simulink model "TrainingTracerVer1"  (R2024a)
settings: Solver=FixedStepAuto  StartTime=0.0  StopTime=inf  RelTol=1e-3  EnableMultiTasking=on
undefined symbols (not defined in the file): bits
libraries: stm32blockslib x30, stm32f4xxblockslib x10, svdutilitieslib x10, simulink x5
settings Model: Creator=niijima  LastModifiedBy=niijima
settings OptimizationCC: EnhancedBackFolding=on  PassReuseOutputArgsAs=Individual arguments  ZeroExternalMemoryAtStartup=off  ZeroInternalMemoryAtStartup=off  MaxStackSize=64  OptimizeBlockOrder=speed  DifferentSizesBufferReuse=on  OptimizationCustomize=off  EfficientTunableParamExpr=on
settings DebuggingCC: ParameterTunabilityLossMsg=error
settings HardwareCC: ProdBitPerPointer=32  ProdBitPerSizeT=32  ProdBitPerPtrDiffT=32  ProdLargestAtomicInteger=Long  ProdLargestAtomicFloat=Double  ProdWordSize=32  ProdLongLongMode=on  ProdHWDeviceType=ARM Compatible->ARM Cortex-M
settings SFSimCC: MATLABDynamicMemAlloc=off
settings RTWCC: Description=Embedded Coder  SystemTargetFile=ert.tlc  HardwareBoard=STM32F3xx Based  TemplateMakefile=ert_default_tmf  Toolchain=GNU Tools for ARM Embedded Processors  BuildConfiguration=Faster Runs
settings CodeAppCC: ForceParamTrailComments=on  IgnoreCustomStorageClasses=off  OperatorAnnotations=on  SimulinkDataObjDesc=on  SFDataObjDesc=on  InsertBlockDesc=on
settings ERTTargetCC: TargetLangStandard=C99 (ISO)  CodeReplacementLibrary=ARM Cortex-M  SupportContinuousTime=on  ExtModeTransport=3  ExtModeStaticAlloc=on  ExtModeStaticAllocSize=2048  ExtModeMexFile=ext_xcp  ExtModeIntrfLevel=Level2 - Open

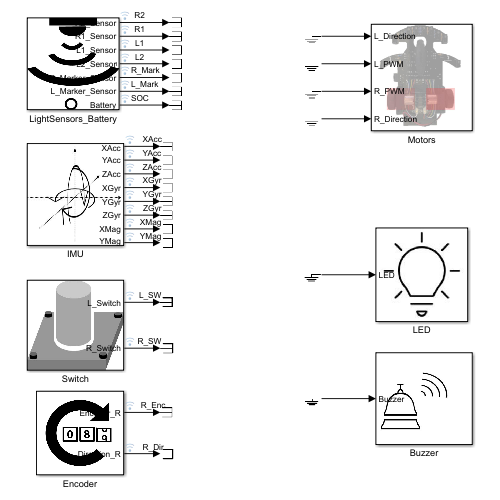
[thumbnail: Simulink's stored preview of the top-level diagram]
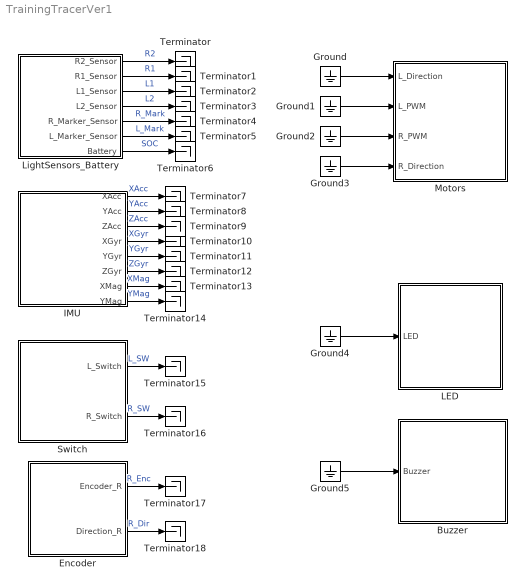
== system TrainingTracerVer1 ==
  Buzzer : Subsystem
      mask Display: image('Buzzer.jpg');
  Encoder : Subsystem
      mask Display: image('Encoder.jpg');
  Ground{,1..5} (6 alike) : Ground
  IMU : Subsystem
      mask Display: image('gyro.jpg');
  LED : Subsystem
      mask Display: image('LED.jpg');
  LightSensors_Battery : Subsystem
      mask Display: image('Sensor.jpg');
  Motors : Subsystem
      mask Display: image('Motor.jpg');
  Switch : Subsystem
      mask Display: image('Switch.jpg');
  Terminator{,1..18} (19 alike) : Terminator
  wires:
  Encoder/2(Direction_R) -> Terminator18/1  "R_Dir"
  Encoder/1(Encoder_R) -> Terminator17/1  "R_Enc"
  IMU/8(YMag) -> Terminator14/1  "YMag"
  IMU/7(XMag) -> Terminator13/1  "XMag"
  IMU/6(ZGyr) -> Terminator12/1  "ZGyr"
  IMU/5(YGyr) -> Terminator11/1  "YGyr"
  IMU/4(XGyr) -> Terminator10/1  "XGyr"
  IMU/3(ZAcc) -> Terminator9/1  "ZAcc"
  IMU/2(YAcc) -> Terminator8/1  "YAcc"
  IMU/1(XAcc) -> Terminator7/1  "XAcc"
  LightSensors_Battery/7(Battery) -> Terminator6/1  "SOC"
  LightSensors_Battery/6(L_Marker_Sensor) -> Terminator5/1  "L_Mark"
  LightSensors_Battery/5(R_Marker_Sensor) -> Terminator4/1  "R_Mark"
  LightSensors_Battery/4(L2_Sensor) -> Terminator3/1  "L2"
  LightSensors_Battery/3(L1_Sensor) -> Terminator2/1  "L1"
  LightSensors_Battery/2(R1_Sensor) -> Terminator1/1  "R1"
  LightSensors_Battery/1(R2_Sensor) -> Terminator/1  "R2"
  Ground3/1 -> Motors/4(R_Direction)
  Ground1/1 -> Motors/2(L_PWM)
  Ground5/1 -> Buzzer/1(Buzzer)
  Ground4/1 -> LED/1(LED)
  Ground2/1 -> Motors/3(R_PWM)
  Ground/1 -> Motors/1(L_Direction)
  Switch/1(L_Switch) -> Terminator15/1  "L_SW"
  Switch/2(R_Switch) -> Terminator16/1  "R_SW"

== system TrainingTracerVer1/Buzzer ==
  Buzzer : Inport
  Buzzer_ : stm32f4xxblockslib/Digital Port Write  PortName=GPIOA  PinNumber=[12]  ReadOperation=off  IOAsArray=on  EnableSimPort=off
      settings: LibrarySourceBlock=stm32f3xxblockslib/Digital Port Write
  wires:
  Buzzer/1 -> Buzzer_/1

== system TrainingTracerVer1/Encoder ==
  Encoder_Left : stm32blockslib/Encoder  Commented=on  TimerModule=TIM20  EnableResetInput=off  OutputDirection=on  SampleTime=-1
      settings: LibrarySourceBlock=stm32f3xxblockslib/Encoder
  Encoder_Right : stm32blockslib/Encoder  TimerModule=TIM2  EnableResetInput=off  OutputDirection=on  SampleTime=-1
      settings: LibrarySourceBlock=stm32f3xxblockslib/Encoder
  Terminator : Terminator
  Terminator1 : Terminator
  Encoder_R : Outport
  Direction_R : Outport  Port=2
  wires:
  Encoder_Right/2 -> Direction_R/1  "Direction_R"
  Encoder_Right/1 -> Encoder_R/1  "Encoder_R"
  Encoder_Left/1 -> Terminator/1  "Encoder_L"
  Encoder_Left/2 -> Terminator1/1  "Direction_L"

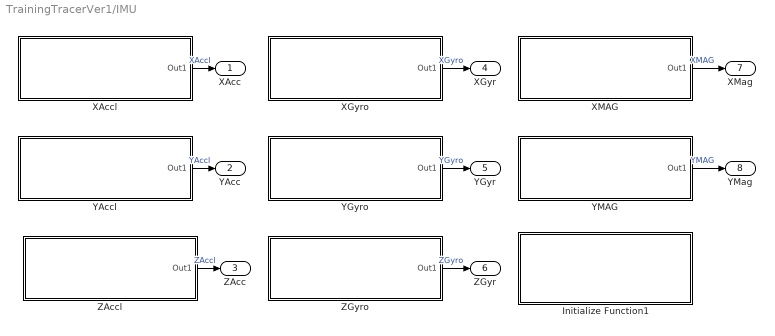
== system TrainingTracerVer1/IMU ==
  Initialize Function1 : Subsystem  TreatAsAtomicUnit=on
  XAccl : Subsystem
  XGyro : Subsystem
  XMAG : Subsystem
  YAccl : Subsystem
  YGyro : Subsystem
  YMAG : Subsystem
  ZAccl : Subsystem
  ZGyro : Subsystem
  XAcc : Outport
  YAcc : Outport  Port=2
  ZAcc : Outport  Port=3
  XGyr : Outport  Port=4
  YGyr : Outport  Port=5
  ZGyr : Outport  Port=6
  XMag : Outport  Port=7
  YMag : Outport  Port=8
  wires:
  XMAG/1(Out1) -> XMag/1  "XMAG"
  YGyro/1(Out1) -> YGyr/1  "YGyro"
  YMAG/1(Out1) -> YMag/1  "YMAG"
  ZGyro/1(Out1) -> ZGyr/1  "ZGyro"
  ZAccl/1(Out1) -> ZAcc/1  "ZAccl"
  XGyro/1(Out1) -> XGyr/1  "XGyro"
  YAccl/1(Out1) -> YAcc/1  "YAccl"
  XAccl/1(Out1) -> XAcc/1  "XAccl"

== system TrainingTracerVer1/LED ==
  LED : Inport
  LED_ : stm32f4xxblockslib/Digital Port Write  PortName=GPIOB  PinNumber=[3]  ReadOperation=off  IOAsArray=on  EnableSimPort=off
      settings: LibrarySourceBlock=stm32f3xxblockslib/Digital Port Write
  wires:
  LED/1 -> LED_/1

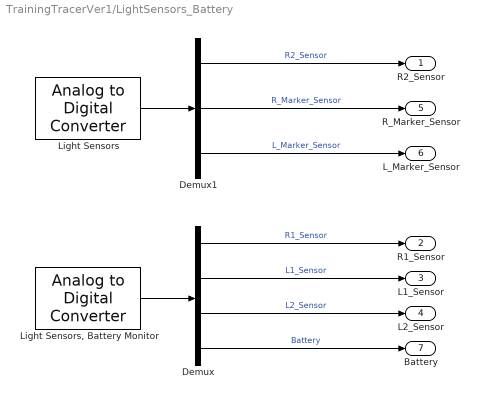
== system TrainingTracerVer1/LightSensors_Battery ==
  Demux : Demux
  Demux1 : Demux  Outputs=3
  Light Sensors : stm32f4xxblockslib/Analog to Digital Converter  ADCModule=ADC1  ConversionGroup=Regular  TriggerMode=Trigger and read  NumberOfConversions=3  EnableBufferConv=off  BufferLength=1  OutputStatus=off  SampleTime=-1  EnableSimPort=off
      settings: LibrarySourceBlock=stm32f3xxblockslib/Analog to Digital Converter
  "Light Sensors, Battery Monitor" : stm32f4xxblockslib/Analog to Digital Converter  ADCModule=ADC2  ConversionGroup=Regular  TriggerMode=Trigger and read  NumberOfConversions=4  EnableBufferConv=off  BufferLength=1  OutputStatus=off  SampleTime=-1  EnableSimPort=off
      settings: LibrarySourceBlock=stm32f3xxblockslib/Analog to Digital Converter
  R2_Sensor : Outport
  R1_Sensor : Outport  Port=2
  L1_Sensor : Outport  Port=3
  L2_Sensor : Outport  Port=4
  R_Marker_Sensor : Outport  Port=5
  L_Marker_Sensor : Outport  Port=6
  Battery : Outport  Port=7
  wires:
  Demux/2 -> L1_Sensor/1  "L1_Sensor"
  "Light Sensors, Battery Monitor"/1 -> Demux/1
  Demux1/1 -> R2_Sensor/1  "R2_Sensor"
  Light Sensors/1 -> Demux1/1
  Demux/3 -> L2_Sensor/1  "L2_Sensor"
  Demux1/3 -> L_Marker_Sensor/1  "L_Marker_Sensor"
  Demux1/2 -> R_Marker_Sensor/1  "R_Marker_Sensor"
  Demux/4 -> Battery/1  "Battery"
  Demux/1 -> R1_Sensor/1  "R1_Sensor"

== system TrainingTracerVer1/Motors ==
  L_Direction : Inport
  L_PWM : Inport  Port=2
  R_PWM : Inport  Port=3
  R_Direction : Inport  Port=4
  Left_Direction : stm32f4xxblockslib/Digital Port Write  PortName=GPIOA  PinNumber=[10]  ReadOperation=off  IOAsArray=on  EnableSimPort=off
      settings: LibrarySourceBlock=stm32f3xxblockslib/Digital Port Write
  Left_PWM : stm32f4xxblockslib/PWM Output  TimerModule=TIM1  DutycycleUnits=Percentage  EnableChannel1=off  EnableChannel2=off  EnableChannel3=off  EnableChannel4=on  EnableCounterInput=off  EnableMainOutputInput=off  EnableFrequencyInput=off  SetRCAfterCE=off  OutputDirection=off  OutputMainOutputEnableStatus=off  SampleTime=0.1  EnableSimPort=off  EnableUpdateEvent=off  EnableCaptureCompare1Event=off  EnableCaptureCompare2Event=off  EnableCaptureCompare3Event=off  EnableCaptureCompare4Event=off  EnableTriggerEvent=off  EnableBreakEvent=off  ProcessorFamily=STM32F3  hoistedMaskSrc=ECSoC/ECSimCodegen/PWM Output
      settings: LibrarySourceBlock=stm32f3xxblockslib/PWM Output
  Right_Direction : stm32f4xxblockslib/Digital Port Write  PortName=GPIOB  PinNumber=[4]  ReadOperation=off  IOAsArray=on  EnableSimPort=off
      settings: LibrarySourceBlock=stm32f3xxblockslib/Digital Port Write
  Right_PWM : stm32f4xxblockslib/PWM Output  TimerModule=TIM17  DutycycleUnits=Percentage  EnableChannel1=on  EnableChannel2=off  EnableChannel3=off  EnableChannel4=off  EnableCounterInput=off  EnableMainOutputInput=off  EnableFrequencyInput=off  SetRCAfterCE=off  OutputDirection=off  OutputMainOutputEnableStatus=off  SampleTime=0.1  EnableSimPort=off  EnableUpdateEvent=off  EnableCaptureCompare1Event=off  EnableCaptureCompare2Event=off  EnableCaptureCompare3Event=off  EnableCaptureCompare4Event=off  EnableTriggerEvent=off  EnableBreakEvent=off  ProcessorFamily=STM32F3  hoistedMaskSrc=ECSoC/ECSimCodegen/PWM Output
      settings: LibrarySourceBlock=stm32f3xxblockslib/PWM Output
  wires:
  R_Direction/1 -> Right_Direction/1
  R_PWM/1 -> Right_PWM/1
  L_Direction/1 -> Left_Direction/1
  L_PWM/1 -> Left_PWM/1

== system TrainingTracerVer1/Switch ==
  L_Switch_ : stm32f4xxblockslib/Digital Port Read  PortName=GPIOF  PinNumber=[0]  ReadOperation=on  IOAsArray=off  SampleTime=-1  EnableSimPort=off
      settings: LibrarySourceBlock=stm32f3xxblockslib/Digital Port Read
  R_Switch_ : stm32f4xxblockslib/Digital Port Read  PortName=GPIOF  PinNumber=[1]  ReadOperation=on  IOAsArray=off  SampleTime=-1  EnableSimPort=off
      settings: LibrarySourceBlock=stm32f3xxblockslib/Digital Port Read
  L_Switch : Outport
  R_Switch : Outport  Port=2
  wires:
  R_Switch_/1 -> R_Switch/1  "R_Switch"
  L_Switch_/1 -> L_Switch/1  "L_Switch"

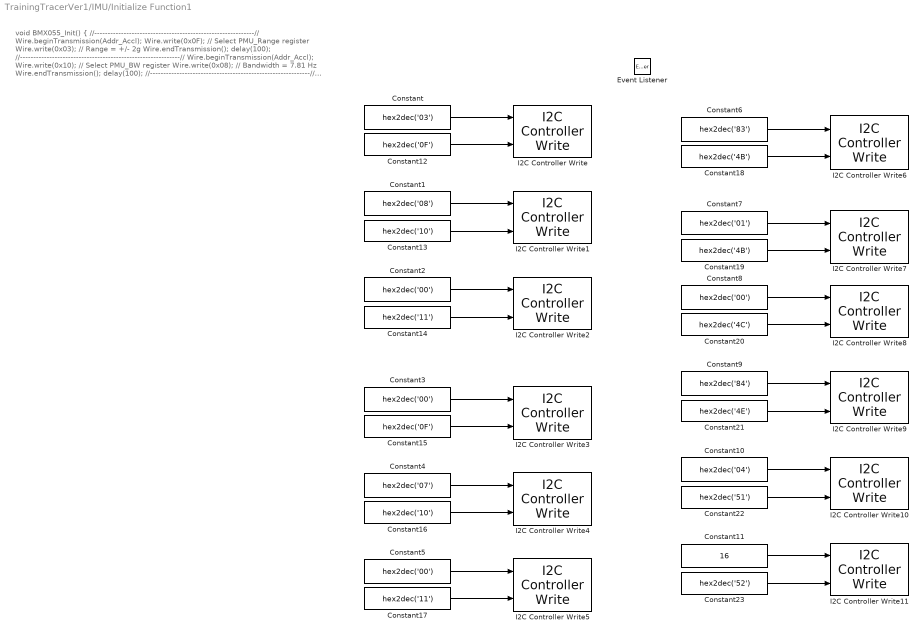
== system TrainingTracerVer1/IMU/Initialize Function1 ==
  note: void BMX055_Init()
      | { //------------------------------------------------------------//
      | Wire.beginTransmission(Addr_Accl);
      | Wire.write(0x0F); // Select PMU_Range register
      | Wire.write(0x03); // Range = +/- 2g
      | Wire.endTransmission();
      | delay(100);
      | //------------------------------------------------------------//
      | Wire.beginTransmission(Addr_Accl);
      | Wire.write(0x10); // Select PMU_BW register
      | Wire.write(0x08); // Bandwidth = 7.81 Hz
      | Wire.endTransmission();
      | delay(100);
      | //------------------------------------------------------------//
      | Wire.beginTransmission(Addr_Accl);
      | Wire.write(0x11); // Select PMU_LPW register
      | Wire.write(0x00); // Normal mode, Sleep duration = 0.5ms
      | Wire.endTransmission();
      | delay(100);
      | //------------------------------------------------------------//
      | Wire.beginTransmission(Addr_Gyro);
      | Wire.write(0x0F); // Select Range register
      | Wire.write(0x00); // Full scale = +/- 2000 degree/s
      | Wire.endTransmission();
      | delay(100);
      | //------------------------------------------------------------//
      | Wire.beginTransmission(Addr_Gyro);
      | Wire.write(0x10); // Select Bandwidth register
      | Wire.write(0x07); // ODR = 100 Hz
      | Wire.endTransmission();
      | delay(100);
      | //------------------------------------------------------------//
      | Wire.beginTransmission(Addr_Gyro);
      | Wire.write(0x11); // Select LPM1 register
      | Wire.write(0x00); // Normal mode, Sleep duration = 2ms
      | Wire.endTransmission();
      | delay(100);
      | //------------------------------------------------------------//
      | Wire.beginTransmission(Addr_Mag);
      | Wire.write(0x4B); // Select Mag register
      | Wire.write(0x83); // Soft reset
      | Wire.endTransmission();
      | delay(100);
      | //------------------------------------------------------------//
      | Wire.beginTransmission(Addr_Mag);
      | Wire.write(0x4B); // Select Mag register
      | Wire.write(0x01); // Soft reset
      | Wire.endTransmission();
      | delay(100);
      | //------------------------------------------------------------//
      | Wire.beginTransmission(Addr_Mag);
      | Wire.write(0x4C); // Select Mag register
      | Wire.write(0x00); // Normal Mode, ODR = 10 Hz
      | Wire.endTransmission();
      | //------------------------------------------------------------//
      | Wire.beginTransmission(Addr_Mag);
      | Wire.write(0x4E); // Select Mag register
      | Wire.write(0x84); // X, Y, Z-Axis enabled
      | Wire.endTransmission();
      | //------------------------------------------------------------//
      | Wire.beginTransmission(Addr_Mag);
      | Wire.write(0x51); // Select Mag register
      | Wire.write(0x04); // No. of Repetitions for X-Y Axis = 9
      | Wire.endTransmission();
      | //------------------------------------------------------------//
      | Wire.beginTransmission(Addr_Mag);
      | Wire.write(0x52); // Select Mag register
      | Wire.write(16); // No. of Repetitions for Z-Axis = 15
      | Wire.endTransmission();}
  Constant : Constant  Value=hex2dec('03')  VectorParams1D=off  OutDataTypeStr=uint8
  Constant1 : Constant  Value=hex2dec('08')  VectorParams1D=off  OutDataTypeStr=uint8
  Constant10 : Constant  Value=hex2dec('04')  VectorParams1D=off  OutDataTypeStr=uint8
  Constant11 : Constant  Value=16  VectorParams1D=off  OutDataTypeStr=uint8
  Constant12 : Constant  Value=hex2dec('0F')  OutDataTypeStr=uint8
  Constant13 : Constant  Value=hex2dec('10')  OutDataTypeStr=uint8
  Constant14 : Constant  Value=hex2dec('11')  OutDataTypeStr=uint8
  Constant15 : Constant  Value=hex2dec('0F')  OutDataTypeStr=uint8
  Constant16 : Constant  Value=hex2dec('10')  OutDataTypeStr=uint8
  Constant17 : Constant  Value=hex2dec('11')  OutDataTypeStr=uint8
  Constant18 : Constant  Value=hex2dec('4B')  OutDataTypeStr=uint8
  Constant19 : Constant  Value=hex2dec('4B')  OutDataTypeStr=uint8
  Constant{2..3,5,8} (4 alike) : Constant  Value=hex2dec('00')  VectorParams1D=off  OutDataTypeStr=uint8
  Constant20 : Constant  Value=hex2dec('4C')  OutDataTypeStr=uint8
  Constant21 : Constant  Value=hex2dec('4E')  OutDataTypeStr=uint8
  Constant22 : Constant  Value=hex2dec('51')  OutDataTypeStr=uint8
  Constant23 : Constant  Value=hex2dec('52')  OutDataTypeStr=uint8
  Constant4 : Constant  Value=hex2dec('07')  VectorParams1D=off  OutDataTypeStr=uint8
  Constant6 : Constant  Value=hex2dec('83')  VectorParams1D=off  OutDataTypeStr=uint8
  Constant7 : Constant  Value=hex2dec('01')  VectorParams1D=off  OutDataTypeStr=uint8
  Constant9 : Constant  Value=hex2dec('84')  VectorParams1D=off  OutDataTypeStr=uint8
  Event Listener : EventListener  DisableCoverage=on  EventName=reset
  I2C Controller Write : stm32blockslib/I2C Controller Write  I2CModule=I2C1  Mode=Controller  AddressingMode=7-bits  PeripheralByteOrder=LittleEndian  OwnPeripheralAddress=uint8(170)  PeripheralAddressVia=Dialog  PeripheralAddress=hex2dec('19')  RegisterAddressMode=on  RegisterAddressVia=Inport  RegisterAddress=hex2dec('0F')  RepeatedStart=off  NoAck=off  OutputStatus=off  BlockMode=Transmit  DataType=uint8  DataLength=1  Timeout=0.1  SampleTime=-1
      settings: LibrarySourceBlock=stm32f4xxblockslib/I2C Controller Write
  I2C Controller Write1 : stm32blockslib/I2C Controller Write  I2CModule=I2C1  Mode=Controller  AddressingMode=7-bits  PeripheralByteOrder=LittleEndian  OwnPeripheralAddress=uint8(170)  PeripheralAddressVia=Dialog  PeripheralAddress=hex2dec('19')  RegisterAddressMode=on  RegisterAddressVia=Inport  RegisterAddress=hex2dec('10')  RepeatedStart=off  NoAck=off  OutputStatus=off  BlockMode=Transmit  DataType=uint8  DataLength=1  Timeout=0.1  SampleTime=-1
      settings: LibrarySourceBlock=stm32f4xxblockslib/I2C Controller Write
  I2C Controller Write10 : stm32blockslib/I2C Controller Write  I2CModule=I2C1  Mode=Controller  AddressingMode=7-bits  PeripheralByteOrder=LittleEndian  OwnPeripheralAddress=uint8(170)  PeripheralAddressVia=Dialog  PeripheralAddress=hex2dec('13')  RegisterAddressMode=on  RegisterAddressVia=Inport  RegisterAddress=hex2dec('51')  RepeatedStart=off  NoAck=off  OutputStatus=off  BlockMode=Transmit  DataType=uint8  DataLength=1  Timeout=0.01  SampleTime=-1
      settings: LibrarySourceBlock=stm32f4xxblockslib/I2C Controller Write
  I2C Controller Write11 : stm32blockslib/I2C Controller Write  I2CModule=I2C1  Mode=Controller  AddressingMode=7-bits  PeripheralByteOrder=LittleEndian  OwnPeripheralAddress=uint8(170)  PeripheralAddressVia=Dialog  PeripheralAddress=hex2dec('13')  RegisterAddressMode=on  RegisterAddressVia=Inport  RegisterAddress=hex2dec('52')  RepeatedStart=off  NoAck=off  OutputStatus=off  BlockMode=Transmit  DataType=uint8  DataLength=1  Timeout=0.01  SampleTime=-1
      settings: LibrarySourceBlock=stm32f4xxblockslib/I2C Controller Write
  I2C Controller Write2 : stm32blockslib/I2C Controller Write  I2CModule=I2C1  Mode=Controller  AddressingMode=7-bits  PeripheralByteOrder=LittleEndian  OwnPeripheralAddress=uint8(170)  PeripheralAddressVia=Dialog  PeripheralAddress=hex2dec('19')  RegisterAddressMode=on  RegisterAddressVia=Inport  RegisterAddress=hex2dec('11')  RepeatedStart=off  NoAck=off  OutputStatus=off  BlockMode=Transmit  DataType=uint8  DataLength=1  Timeout=0.1  SampleTime=-1
      settings: LibrarySourceBlock=stm32f4xxblockslib/I2C Controller Write
  I2C Controller Write3 : stm32blockslib/I2C Controller Write  I2CModule=I2C1  Mode=Controller  AddressingMode=7-bits  PeripheralByteOrder=LittleEndian  OwnPeripheralAddress=uint8(170)  PeripheralAddressVia=Dialog  PeripheralAddress=hex2dec('69')  RegisterAddressMode=on  RegisterAddressVia=Inport  RegisterAddress=hex2dec('0F')  RepeatedStart=off  NoAck=off  OutputStatus=off  BlockMode=Transmit  DataType=uint8  DataLength=1  Timeout=0.1  SampleTime=-1
      settings: LibrarySourceBlock=stm32f4xxblockslib/I2C Controller Write
  I2C Controller Write4 : stm32blockslib/I2C Controller Write  I2CModule=I2C1  Mode=Controller  AddressingMode=7-bits  PeripheralByteOrder=LittleEndian  OwnPeripheralAddress=uint8(170)  PeripheralAddressVia=Dialog  PeripheralAddress=hex2dec('69')  RegisterAddressMode=on  RegisterAddressVia=Inport  RegisterAddress=hex2dec('10')  RepeatedStart=off  NoAck=off  OutputStatus=off  BlockMode=Transmit  DataType=uint8  DataLength=1  Timeout=0.1  SampleTime=-1
      settings: LibrarySourceBlock=stm32f4xxblockslib/I2C Controller Write
  I2C Controller Write5 : stm32blockslib/I2C Controller Write  I2CModule=I2C1  Mode=Controller  AddressingMode=7-bits  PeripheralByteOrder=LittleEndian  OwnPeripheralAddress=uint8(170)  PeripheralAddressVia=Dialog  PeripheralAddress=hex2dec('69')  RegisterAddressMode=on  RegisterAddressVia=Inport  RegisterAddress=hex2dec('11')  RepeatedStart=off  NoAck=off  OutputStatus=off  BlockMode=Transmit  DataType=uint8  DataLength=1  Timeout=0.1  SampleTime=-1
      settings: LibrarySourceBlock=stm32f4xxblockslib/I2C Controller Write
  I2C Controller Write6 : stm32blockslib/I2C Controller Write  I2CModule=I2C1  Mode=Controller  AddressingMode=7-bits  PeripheralByteOrder=LittleEndian  OwnPeripheralAddress=uint8(170)  PeripheralAddressVia=Dialog  PeripheralAddress=hex2dec('13')  RegisterAddressMode=on  RegisterAddressVia=Inport  RegisterAddress=hex2dec('4B')  RepeatedStart=off  NoAck=off  OutputStatus=off  BlockMode=Transmit  DataType=uint8  DataLength=1  Timeout=0.1  SampleTime=-1
      settings: LibrarySourceBlock=stm32f4xxblockslib/I2C Controller Write
  I2C Controller Write7 : stm32blockslib/I2C Controller Write  I2CModule=I2C1  Mode=Controller  AddressingMode=7-bits  PeripheralByteOrder=LittleEndian  OwnPeripheralAddress=uint8(170)  PeripheralAddressVia=Dialog  PeripheralAddress=hex2dec('13')  RegisterAddressMode=on  RegisterAddressVia=Inport  RegisterAddress=hex2dec('4B')  RepeatedStart=off  NoAck=off  OutputStatus=off  BlockMode=Transmit  DataType=uint8  DataLength=1  Timeout=0.1  SampleTime=-1
      settings: LibrarySourceBlock=stm32f4xxblockslib/I2C Controller Write
  I2C Controller Write8 : stm32blockslib/I2C Controller Write  I2CModule=I2C1  Mode=Controller  AddressingMode=7-bits  PeripheralByteOrder=LittleEndian  OwnPeripheralAddress=uint8(170)  PeripheralAddressVia=Dialog  PeripheralAddress=hex2dec('13')  RegisterAddressMode=on  RegisterAddressVia=Inport  RegisterAddress=hex2dec('4C')  RepeatedStart=off  NoAck=off  OutputStatus=off  BlockMode=Transmit  DataType=uint8  DataLength=1  Timeout=0.01  SampleTime=-1
      settings: LibrarySourceBlock=stm32f4xxblockslib/I2C Controller Write
  I2C Controller Write9 : stm32blockslib/I2C Controller Write  I2CModule=I2C1  Mode=Controller  AddressingMode=7-bits  PeripheralByteOrder=LittleEndian  OwnPeripheralAddress=uint8(170)  PeripheralAddressVia=Dialog  PeripheralAddress=hex2dec('13')  RegisterAddressMode=on  RegisterAddressVia=Inport  RegisterAddress=hex2dec('4E')  RepeatedStart=off  NoAck=off  OutputStatus=off  BlockMode=Transmit  DataType=uint8  DataLength=1  Timeout=0.01  SampleTime=-1
      settings: LibrarySourceBlock=stm32f4xxblockslib/I2C Controller Write
  wires:
  Constant/1 -> I2C Controller Write/1
  Constant1/1 -> I2C Controller Write1/1
  Constant2/1 -> I2C Controller Write2/1
  Constant5/1 -> I2C Controller Write5/1
  Constant4/1 -> I2C Controller Write4/1
  Constant3/1 -> I2C Controller Write3/1
  Constant6/1 -> I2C Controller Write6/1
  Constant7/1 -> I2C Controller Write7/1
  Constant8/1 -> I2C Controller Write8/1
  Constant9/1 -> I2C Controller Write9/1
  Constant10/1 -> I2C Controller Write10/1
  Constant11/1 -> I2C Controller Write11/1
  Constant12/1 -> I2C Controller Write/2
  Constant13/1 -> I2C Controller Write1/2
  Constant14/1 -> I2C Controller Write2/2
  Constant15/1 -> I2C Controller Write3/2
  Constant16/1 -> I2C Controller Write4/2
  Constant17/1 -> I2C Controller Write5/2
  Constant18/1 -> I2C Controller Write6/2
  Constant19/1 -> I2C Controller Write7/2
  Constant20/1 -> I2C Controller Write8/2
  Constant21/1 -> I2C Controller Write9/2
  Constant22/1 -> I2C Controller Write10/2
  Constant23/1 -> I2C Controller Write11/2

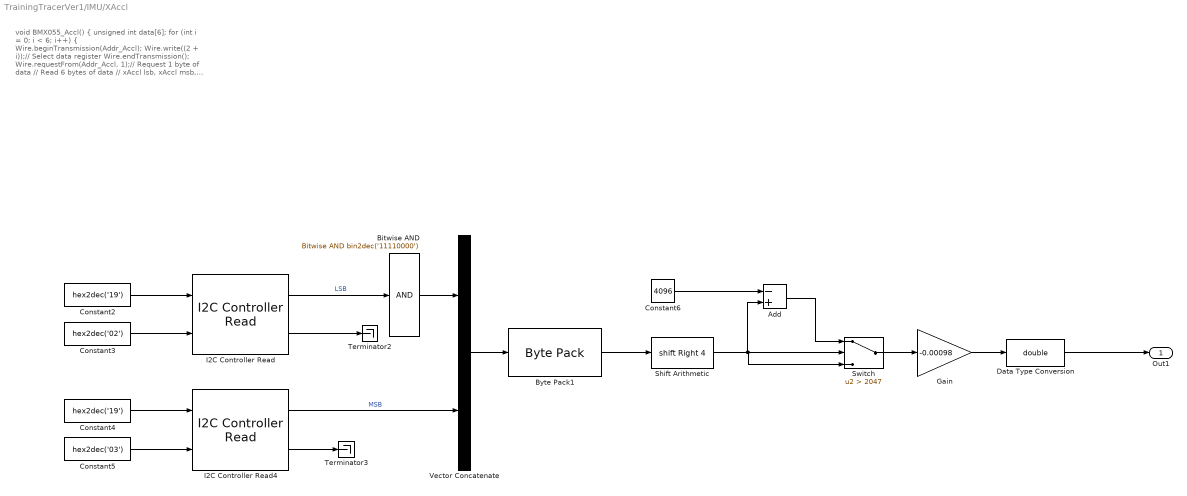
== system TrainingTracerVer1/IMU/XAccl ==
  note: void BMX055_Accl()
      | {
      | unsigned int data[6];
      | for (int i = 0; i < 6; i++)
      | {
      | Wire.beginTransmission(Addr_Accl);
      | Wire.write((2 + i));// Select data register
      | Wire.endTransmission();
      | Wire.requestFrom(Addr_Accl, 1);// Request 1 byte of data
      | // Read 6 bytes of data
      | // xAccl lsb, xAccl msb, yAccl lsb, yAccl msb, zAccl lsb, zAccl msb
      | if (Wire.available() == 1)
      | data[i] = Wire.read();
      | }
      | // Convert the data to 12-bits
      | xAccl = ((data[1] * 256) + (data[0] & 0xF0)) / 16;
      | if (xAccl > 2047) xAccl -= 4096;
      | xAccl = xAccl * 0.00098; // range = +/-2g
      | }
  Add : Sum  Inputs=-+
  Bitwise AND : simulink/Logic and Bit Operations/Bitwise Operator  logicop=AND  UseBitMask=on  BitMask=bin2dec('11110000')  BitMaskRealWorld=Stored Integer
      settings: LibrarySourceBlock=|
      | simulink/Quick Insert/Logic and Bit
      | Operations/Bitwise AND
  Byte Pack1 : svdutilitieslib/Byte Pack  maskPackedDataType=uint16  datatypes={'uint8'}  byteAlign=1  blockPlatform=arduinoert
      settings: LibrarySourceBlock=mcblib/Signal Management/Byte Pack
  Constant2 : Constant  Value=hex2dec('19')  OutDataTypeStr=uint8
  Constant3 : Constant  Value=hex2dec('02')  OutDataTypeStr=uint8
  Constant4 : Constant  Value=hex2dec('19')  OutDataTypeStr=uint8
  Constant5 : Constant  Value=hex2dec('03')  OutDataTypeStr=uint8
  Constant6 : Constant  Value=4096
  Data Type Conversion : DataTypeConversion  OutDataTypeStr=double  SaturateOnIntegerOverflow=off  RndMeth=Floor
  Gain : Gain  Gain=-0.00098
  I2C Controller Read : stm32blockslib/I2C Controller Read  I2CModule=I2C1  Mode=Controller  AddressingMode=7-bits  PeripheralByteOrder=LittleEndian  OwnPeripheralAddress=uint8(170)  PeripheralAddressVia=Inport  PeripheralAddress=0x19  RegisterAddressMode=on  RegisterAddressVia=Inport  RegisterAddress=0x02  RepeatedStart=off  NoAck=off  OutputStatus=on  BlockMode=Receive  DataType=uint8  DataLength=1  Timeout=0.1  SampleTime=-1
      settings: LibrarySourceBlock=stm32f4xxblockslib/I2C Controller Read
  I2C Controller Read4 : stm32blockslib/I2C Controller Read  I2CModule=I2C1  Mode=Controller  AddressingMode=7-bits  PeripheralByteOrder=LittleEndian  OwnPeripheralAddress=uint8(170)  PeripheralAddressVia=Inport  PeripheralAddress=0x19  RegisterAddressMode=on  RegisterAddressVia=Inport  RegisterAddress=0x02  RepeatedStart=off  NoAck=off  OutputStatus=on  BlockMode=Receive  DataType=uint8  DataLength=1  Timeout=0.1  SampleTime=-1
      settings: LibrarySourceBlock=stm32f4xxblockslib/I2C Controller Read
  Shift Arithmetic : ArithShift  BitShiftNumber=4  BitShiftDirection=Right
  Switch : Switch  Criteria=u2 > Threshold  Threshold=2047  SaturateOnIntegerOverflow=off  InputSameDT=off
  Terminator2 : Terminator
  Terminator3 : Terminator
  Vector Concatenate : Concatenate
  Out1 : Outport
  wires:
  Constant3/1 -> I2C Controller Read/2
  Add/1 -> Switch/1
  Constant4/1 -> I2C Controller Read4/1
  Byte Pack1/1 -> Shift Arithmetic/1
  Gain/1 -> Data Type Conversion/1
  I2C Controller Read/2 -> Terminator2/1
  Constant2/1 -> I2C Controller Read/1
  Shift Arithmetic/1 -> Switch/2, Switch/3, Add/2
  Bitwise AND/1 -> Vector Concatenate/1
  Constant6/1 -> Add/1
  I2C Controller Read4/2 -> Terminator3/1
  I2C Controller Read4/1 -> Vector Concatenate/2  "MSB"
  Constant5/1 -> I2C Controller Read4/2
  Switch/1 -> Gain/1
  I2C Controller Read/1 -> Bitwise AND/1  "LSB"
  Vector Concatenate/1 -> Byte Pack1/1
  Data Type Conversion/1 -> Out1/1

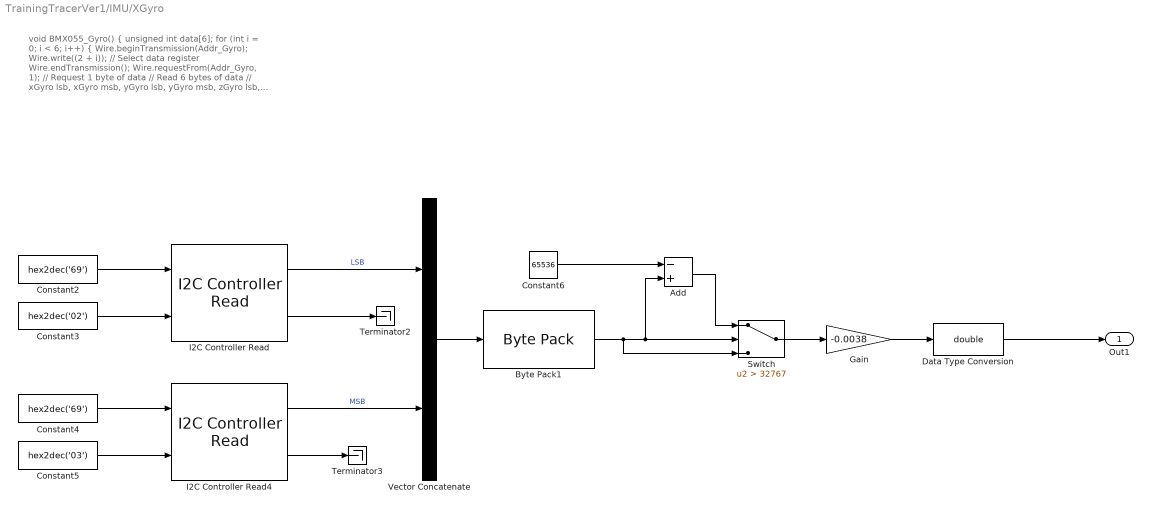
== system TrainingTracerVer1/IMU/XGyro ==
  note: void BMX055_Gyro()
      | {
      | unsigned int data[6];
      | for (int i = 0; i < 6; i++)
      | {
      | Wire.beginTransmission(Addr_Gyro);
      | Wire.write((2 + i)); // Select data register
      | Wire.endTransmission();
      | Wire.requestFrom(Addr_Gyro, 1); // Request 1 byte of data
      | // Read 6 bytes of data
      | // xGyro lsb, xGyro msb, yGyro lsb, yGyro msb, zGyro lsb, zGyro msb
      | if (Wire.available() == 1)
      | data[i] = Wire.read();
      | }
      | // Convert the data
      | xGyro = (data[1] * 256) + data[0];
      | if (xGyro > 32767) xGyro -= 65536;
      | }
  Add : Sum  Inputs=-+
  Byte Pack1 : svdutilitieslib/Byte Pack  maskPackedDataType=uint16  datatypes={'uint8'}  byteAlign=1  blockPlatform=arduinoert
      settings: LibrarySourceBlock=mcblib/Signal Management/Byte Pack
  Constant2 : Constant  Value=hex2dec('69')  OutDataTypeStr=uint8
  Constant3 : Constant  Value=hex2dec('02')  OutDataTypeStr=uint8
  Constant4 : Constant  Value=hex2dec('69')  OutDataTypeStr=uint8
  Constant5 : Constant  Value=hex2dec('03')  OutDataTypeStr=uint8
  Constant6 : Constant  Value=65536
  Data Type Conversion : DataTypeConversion  OutDataTypeStr=double  SaturateOnIntegerOverflow=off  RndMeth=Floor
  Gain : Gain  Gain=-0.0038
  I2C Controller Read : stm32blockslib/I2C Controller Read  I2CModule=I2C1  Mode=Controller  AddressingMode=7-bits  PeripheralByteOrder=LittleEndian  OwnPeripheralAddress=uint8(170)  PeripheralAddressVia=Inport  PeripheralAddress=0x19  RegisterAddressMode=on  RegisterAddressVia=Inport  RegisterAddress=0x02  RepeatedStart=off  NoAck=off  OutputStatus=on  BlockMode=Receive  DataType=uint8  DataLength=1  Timeout=0.1  SampleTime=-1
      settings: LibrarySourceBlock=stm32f4xxblockslib/I2C Controller Read
  I2C Controller Read4 : stm32blockslib/I2C Controller Read  I2CModule=I2C1  Mode=Controller  AddressingMode=7-bits  PeripheralByteOrder=LittleEndian  OwnPeripheralAddress=uint8(170)  PeripheralAddressVia=Inport  PeripheralAddress=0x19  RegisterAddressMode=on  RegisterAddressVia=Inport  RegisterAddress=0x02  RepeatedStart=off  NoAck=off  OutputStatus=on  BlockMode=Receive  DataType=uint8  DataLength=1  Timeout=0.1  SampleTime=-1
      settings: LibrarySourceBlock=stm32f4xxblockslib/I2C Controller Read
  Switch : Switch  Criteria=u2 > Threshold  Threshold=32767  SaturateOnIntegerOverflow=off  InputSameDT=off
  Terminator2 : Terminator
  Terminator3 : Terminator
  Vector Concatenate : Concatenate
  Out1 : Outport
  wires:
  Constant3/1 -> I2C Controller Read/2
  Add/1 -> Switch/1
  Constant4/1 -> I2C Controller Read4/1
  Gain/1 -> Data Type Conversion/1
  I2C Controller Read/2 -> Terminator2/1
  Constant2/1 -> I2C Controller Read/1
  Byte Pack1/1 -> Switch/2, Add/2, Switch/3
  Constant6/1 -> Add/1
  I2C Controller Read4/2 -> Terminator3/1
  I2C Controller Read4/1 -> Vector Concatenate/2  "MSB"
  Constant5/1 -> I2C Controller Read4/2
  Switch/1 -> Gain/1
  I2C Controller Read/1 -> Vector Concatenate/1  "LSB"
  Vector Concatenate/1 -> Byte Pack1/1
  Data Type Conversion/1 -> Out1/1

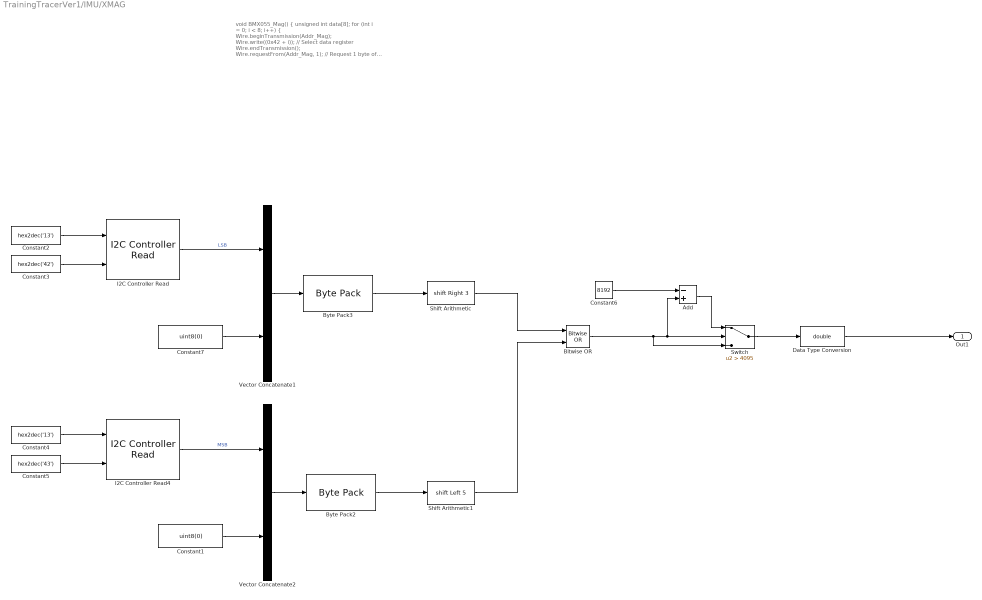
== system TrainingTracerVer1/IMU/XMAG ==
  note: void BMX055_Mag()
      | {
      | unsigned int data[8];
      | for (int i = 0; i < 8; i++)
      | {
      | Wire.beginTransmission(Addr_Mag);
      | Wire.write((0x42 + i)); // Select data register
      | Wire.endTransmission();
      | Wire.requestFrom(Addr_Mag, 1); // Request 1 byte of data
      | // Read 6 bytes of data
      | // xMag lsb, xMag msb, yMag lsb, yMag msb, zMag lsb, zMag msb
      | if (Wire.available() == 1)
      | data[i] = Wire.read();
      | }
      | // Convert the data
      | xMag = ((data[1] <<5) | (data[0]>>3));
      | if (xMag > 4095) xMag -= 8192;
      | }
  Add : Sum  Inputs=-+
  Bitwise OR : simulink/Logic and Bit Operations/Bitwise Operator  logicop=OR  UseBitMask=off  NumInputPorts=2  BitMask=bin2dec('11011001')  BitMaskRealWorld=Stored Integer
      settings: LibrarySourceBlock=|
      | simulink/Quick Insert/Logic and Bit
      | Operations/Bitwise OR
  Byte Pack2 : svdutilitieslib/Byte Pack  maskPackedDataType=uint16  datatypes={'uint8'}  byteAlign=1  blockPlatform=arduinoert
      settings: LibrarySourceBlock=mcblib/Signal Management/Byte Pack
  Byte Pack3 : svdutilitieslib/Byte Pack  maskPackedDataType=uint16  datatypes={'uint8'}  byteAlign=1  blockPlatform=arduinoert
      settings: LibrarySourceBlock=mcblib/Signal Management/Byte Pack
  Constant1 : Constant  Value=uint8(0)
  Constant2 : Constant  Value=hex2dec('13')  OutDataTypeStr=uint8
  Constant3 : Constant  Value=hex2dec('42')  OutDataTypeStr=uint8
  Constant4 : Constant  Value=hex2dec('13')  OutDataTypeStr=uint8
  Constant5 : Constant  Value=hex2dec('43')  OutDataTypeStr=uint8
  Constant6 : Constant  Value=8192
  Constant7 : Constant  Value=uint8(0)
  Data Type Conversion : DataTypeConversion  OutDataTypeStr=double  SaturateOnIntegerOverflow=off  RndMeth=Floor
  I2C Controller Read : stm32blockslib/I2C Controller Read  I2CModule=I2C1  Mode=Controller  AddressingMode=7-bits  PeripheralByteOrder=LittleEndian  OwnPeripheralAddress=uint8(170)  PeripheralAddressVia=Inport  PeripheralAddress=0x19  RegisterAddressMode=on  RegisterAddressVia=Inport  RegisterAddress=0x02  RepeatedStart=off  NoAck=off  OutputStatus=off  BlockMode=Receive  DataType=uint8  DataLength=1  Timeout=0.001  SampleTime=-1
      settings: LibrarySourceBlock=stm32f4xxblockslib/I2C Controller Read
  I2C Controller Read4 : stm32blockslib/I2C Controller Read  I2CModule=I2C1  Mode=Controller  AddressingMode=7-bits  PeripheralByteOrder=LittleEndian  OwnPeripheralAddress=uint8(170)  PeripheralAddressVia=Inport  PeripheralAddress=0x19  RegisterAddressMode=on  RegisterAddressVia=Inport  RegisterAddress=0x02  RepeatedStart=off  NoAck=off  OutputStatus=off  BlockMode=Receive  DataType=uint8  DataLength=1  Timeout=0.001  SampleTime=-1
      settings: LibrarySourceBlock=stm32f4xxblockslib/I2C Controller Read
  Shift Arithmetic : ArithShift  BitShiftNumber=3  BitShiftDirection=Right
  Shift Arithmetic1 : ArithShift  BitShiftNumber=5  BitShiftDirection=Left
  Switch : Switch  Criteria=u2 > Threshold  Threshold=4095  SaturateOnIntegerOverflow=off  InputSameDT=off
  Vector Concatenate1 : Concatenate
  Vector Concatenate2 : Concatenate
  Out1 : Outport
  wires:
  Constant3/1 -> I2C Controller Read/2
  Add/1 -> Switch/1
  Constant4/1 -> I2C Controller Read4/1
  Switch/1 -> Data Type Conversion/1
  Constant2/1 -> I2C Controller Read/1
  Bitwise OR/1 -> Switch/2, Add/2, Switch/3
  Constant6/1 -> Add/1
  I2C Controller Read4/1 -> Vector Concatenate2/1  "MSB"
  Constant5/1 -> I2C Controller Read4/2
  I2C Controller Read/1 -> Vector Concatenate1/1  "LSB"
  Data Type Conversion/1 -> Out1/1
  Shift Arithmetic/1 -> Bitwise OR/1
  Shift Arithmetic1/1 -> Bitwise OR/2
  Constant1/1 -> Vector Concatenate2/2
  Vector Concatenate2/1 -> Byte Pack2/1
  Vector Concatenate1/1 -> Byte Pack3/1
  Constant7/1 -> Vector Concatenate1/2
  Byte Pack3/1 -> Shift Arithmetic/1
  Byte Pack2/1 -> Shift Arithmetic1/1

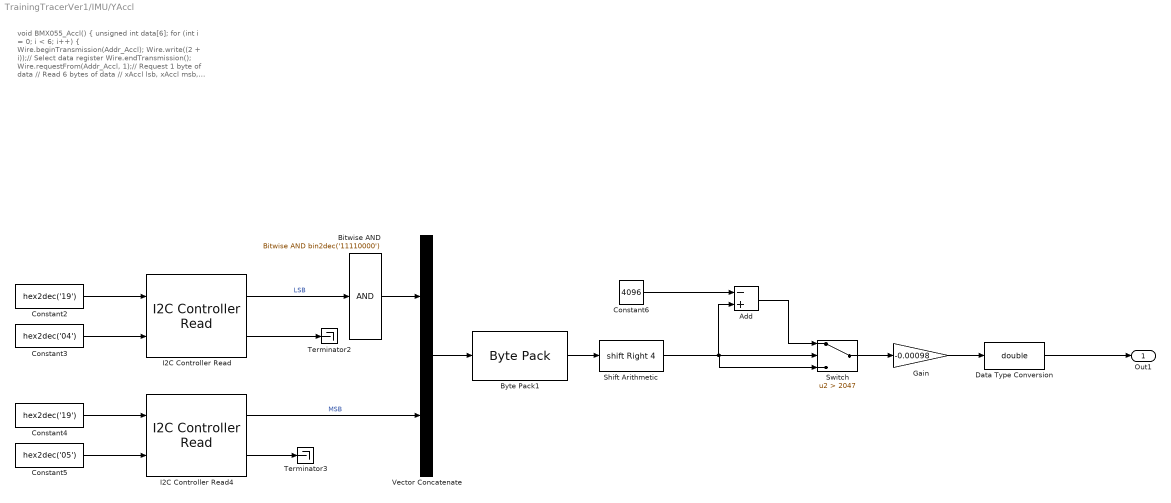
== system TrainingTracerVer1/IMU/YAccl ==
  note: void BMX055_Accl()
      | {
      | unsigned int data[6];
      | for (int i = 0; i < 6; i++)
      | {
      | Wire.beginTransmission(Addr_Accl);
      | Wire.write((2 + i));// Select data register
      | Wire.endTransmission();
      | Wire.requestFrom(Addr_Accl, 1);// Request 1 byte of data
      | // Read 6 bytes of data
      | // xAccl lsb, xAccl msb, yAccl lsb, yAccl msb, zAccl lsb, zAccl msb
      | if (Wire.available() == 1)
      | data[i] = Wire.read();
      | }
      | // Convert the data to 12-bits
      | yAccl = ((data[3] * 256) + (data[2] & 0xF0)) / 16;
      | if (yAccl > 2047) yAccl -= 4096;
      | yAccl = yAccl * 0.00098; // range = +/-2g
      | }
  Add : Sum  Inputs=-+
  Bitwise AND : simulink/Logic and Bit Operations/Bitwise Operator  logicop=AND  UseBitMask=on  BitMask=bin2dec('11110000')  BitMaskRealWorld=Stored Integer
      settings: LibrarySourceBlock=|
      | simulink/Quick Insert/Logic and Bit
      | Operations/Bitwise AND
  Byte Pack1 : svdutilitieslib/Byte Pack  maskPackedDataType=uint16  datatypes={'uint8'}  byteAlign=1  blockPlatform=arduinoert
      settings: LibrarySourceBlock=mcblib/Signal Management/Byte Pack
  Constant2 : Constant  Value=hex2dec('19')  OutDataTypeStr=uint8
  Constant3 : Constant  Value=hex2dec('04')  OutDataTypeStr=uint8
  Constant4 : Constant  Value=hex2dec('19')  OutDataTypeStr=uint8
  Constant5 : Constant  Value=hex2dec('05')  OutDataTypeStr=uint8
  Constant6 : Constant  Value=4096
  Data Type Conversion : DataTypeConversion  OutDataTypeStr=double  SaturateOnIntegerOverflow=off  RndMeth=Floor
  Gain : Gain  Gain=-0.00098
  I2C Controller Read : stm32blockslib/I2C Controller Read  I2CModule=I2C1  Mode=Controller  AddressingMode=7-bits  PeripheralByteOrder=LittleEndian  OwnPeripheralAddress=uint8(170)  PeripheralAddressVia=Inport  PeripheralAddress=0x19  RegisterAddressMode=on  RegisterAddressVia=Inport  RegisterAddress=0x02  RepeatedStart=off  NoAck=off  OutputStatus=on  BlockMode=Receive  DataType=uint8  DataLength=1  Timeout=0.1  SampleTime=-1
      settings: LibrarySourceBlock=stm32f4xxblockslib/I2C Controller Read
  I2C Controller Read4 : stm32blockslib/I2C Controller Read  I2CModule=I2C1  Mode=Controller  AddressingMode=7-bits  PeripheralByteOrder=LittleEndian  OwnPeripheralAddress=uint8(170)  PeripheralAddressVia=Inport  PeripheralAddress=0x19  RegisterAddressMode=on  RegisterAddressVia=Inport  RegisterAddress=0x02  RepeatedStart=off  NoAck=off  OutputStatus=on  BlockMode=Receive  DataType=uint8  DataLength=1  Timeout=0.1  SampleTime=-1
      settings: LibrarySourceBlock=stm32f4xxblockslib/I2C Controller Read
  Shift Arithmetic : ArithShift  BitShiftNumber=4  BitShiftDirection=Right
  Switch : Switch  Criteria=u2 > Threshold  Threshold=2047  SaturateOnIntegerOverflow=off  InputSameDT=off
  Terminator2 : Terminator
  Terminator3 : Terminator
  Vector Concatenate : Concatenate
  Out1 : Outport
  wires:
  Constant3/1 -> I2C Controller Read/2
  Add/1 -> Switch/1
  Constant4/1 -> I2C Controller Read4/1
  Byte Pack1/1 -> Shift Arithmetic/1
  Gain/1 -> Data Type Conversion/1
  I2C Controller Read/2 -> Terminator2/1
  Constant2/1 -> I2C Controller Read/1
  Shift Arithmetic/1 -> Switch/2, Switch/3, Add/2
  Bitwise AND/1 -> Vector Concatenate/1
  Constant6/1 -> Add/1
  I2C Controller Read4/2 -> Terminator3/1
  I2C Controller Read4/1 -> Vector Concatenate/2  "MSB"
  Constant5/1 -> I2C Controller Read4/2
  Switch/1 -> Gain/1
  I2C Controller Read/1 -> Bitwise AND/1  "LSB"
  Vector Concatenate/1 -> Byte Pack1/1
  Data Type Conversion/1 -> Out1/1

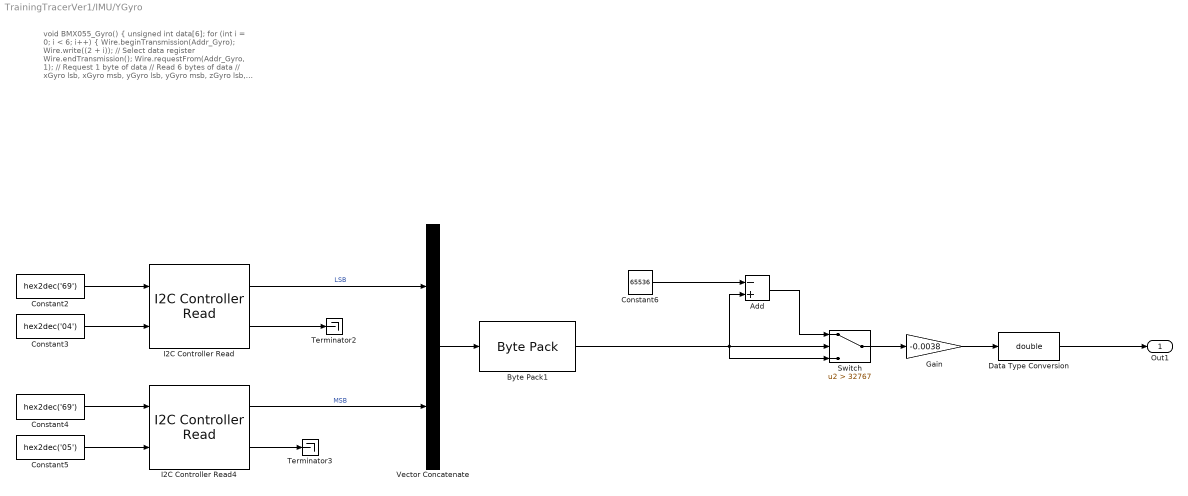
== system TrainingTracerVer1/IMU/YGyro ==
  note: void BMX055_Gyro()
      | {
      | unsigned int data[6];
      | for (int i = 0; i < 6; i++)
      | {
      | Wire.beginTransmission(Addr_Gyro);
      | Wire.write((2 + i)); // Select data register
      | Wire.endTransmission();
      | Wire.requestFrom(Addr_Gyro, 1); // Request 1 byte of data
      | // Read 6 bytes of data
      | // xGyro lsb, xGyro msb, yGyro lsb, yGyro msb, zGyro lsb, zGyro msb
      | if (Wire.available() == 1)
      | data[i] = Wire.read();
      | }
      | // Convert the data
      | yGyro = (data[3] * 256) + data[2];
      | if (yGyro > 32767) yGyro -= 65536;
      | yGyro = yGyro * 0.0038; // Full scale = +/- 125 degree/s
      | }
  Add : Sum  Inputs=-+
  Byte Pack1 : svdutilitieslib/Byte Pack  maskPackedDataType=uint16  datatypes={'uint8'}  byteAlign=1  blockPlatform=arduinoert
      settings: LibrarySourceBlock=mcblib/Signal Management/Byte Pack
  Constant2 : Constant  Value=hex2dec('69')  OutDataTypeStr=uint8
  Constant3 : Constant  Value=hex2dec('04')  OutDataTypeStr=uint8
  Constant4 : Constant  Value=hex2dec('69')  OutDataTypeStr=uint8
  Constant5 : Constant  Value=hex2dec('05')  OutDataTypeStr=uint8
  Constant6 : Constant  Value=65536
  Data Type Conversion : DataTypeConversion  OutDataTypeStr=double  SaturateOnIntegerOverflow=off  RndMeth=Floor
  Gain : Gain  Gain=-0.0038
  I2C Controller Read : stm32blockslib/I2C Controller Read  I2CModule=I2C1  Mode=Controller  AddressingMode=7-bits  PeripheralByteOrder=LittleEndian  OwnPeripheralAddress=uint8(170)  PeripheralAddressVia=Inport  PeripheralAddress=0x19  RegisterAddressMode=on  RegisterAddressVia=Inport  RegisterAddress=0x02  RepeatedStart=off  NoAck=off  OutputStatus=on  BlockMode=Receive  DataType=uint8  DataLength=1  Timeout=0.1  SampleTime=-1
      settings: LibrarySourceBlock=stm32f4xxblockslib/I2C Controller Read
  I2C Controller Read4 : stm32blockslib/I2C Controller Read  I2CModule=I2C1  Mode=Controller  AddressingMode=7-bits  PeripheralByteOrder=LittleEndian  OwnPeripheralAddress=uint8(170)  PeripheralAddressVia=Inport  PeripheralAddress=0x19  RegisterAddressMode=on  RegisterAddressVia=Inport  RegisterAddress=0x02  RepeatedStart=off  NoAck=off  OutputStatus=on  BlockMode=Receive  DataType=uint8  DataLength=1  Timeout=0.1  SampleTime=-1
      settings: LibrarySourceBlock=stm32f4xxblockslib/I2C Controller Read
  Switch : Switch  Criteria=u2 > Threshold  Threshold=32767  SaturateOnIntegerOverflow=off  InputSameDT=off
  Terminator2 : Terminator
  Terminator3 : Terminator
  Vector Concatenate : Concatenate
  Out1 : Outport
  wires:
  Constant3/1 -> I2C Controller Read/2
  Add/1 -> Switch/1
  Constant4/1 -> I2C Controller Read4/1
  Gain/1 -> Data Type Conversion/1
  I2C Controller Read/2 -> Terminator2/1
  Constant2/1 -> I2C Controller Read/1
  Byte Pack1/1 -> Switch/2, Switch/3, Add/2
  Constant6/1 -> Add/1
  I2C Controller Read4/2 -> Terminator3/1
  I2C Controller Read4/1 -> Vector Concatenate/2  "MSB"
  Constant5/1 -> I2C Controller Read4/2
  Switch/1 -> Gain/1
  I2C Controller Read/1 -> Vector Concatenate/1  "LSB"
  Vector Concatenate/1 -> Byte Pack1/1
  Data Type Conversion/1 -> Out1/1

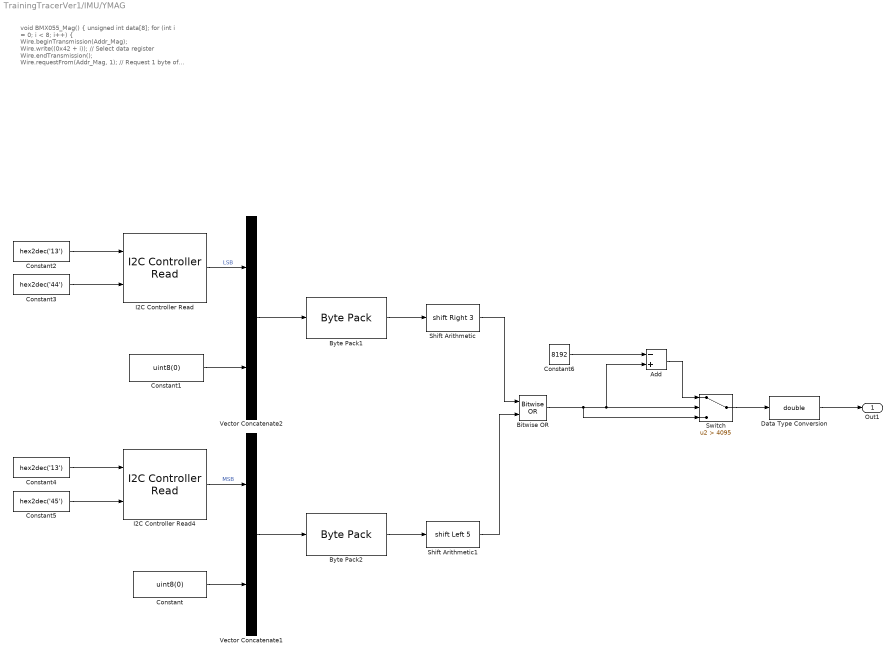
== system TrainingTracerVer1/IMU/YMAG ==
  note: void BMX055_Mag()
      | {
      | unsigned int data[8];
      | for (int i = 0; i < 8; i++)
      | {
      | Wire.beginTransmission(Addr_Mag);
      | Wire.write((0x42 + i)); // Select data register
      | Wire.endTransmission();
      | Wire.requestFrom(Addr_Mag, 1); // Request 1 byte of data
      | // Read 6 bytes of data
      | // xMag lsb, xMag msb, yMag lsb, yMag msb, zMag lsb, zMag msb
      | if (Wire.available() == 1)
      | data[i] = Wire.read();
      | }
      | // Convert the data
      | yMag = ((data[3] <<5) | (data[2]>>3));
      | if (yMag > 4095) yMag -= 8192;
      | }
  Add : Sum  Inputs=-+
  Bitwise OR : simulink/Logic and Bit Operations/Bitwise Operator  logicop=OR  UseBitMask=off  NumInputPorts=2  BitMask=bin2dec('11011001')  BitMaskRealWorld=Stored Integer
      settings: LibrarySourceBlock=|
      | simulink/Quick Insert/Logic and Bit
      | Operations/Bitwise OR
  Byte Pack1 : svdutilitieslib/Byte Pack  maskPackedDataType=uint16  datatypes={'uint8'}  byteAlign=1  blockPlatform=arduinoert
      settings: LibrarySourceBlock=mcblib/Signal Management/Byte Pack
  Byte Pack2 : svdutilitieslib/Byte Pack  maskPackedDataType=uint16  datatypes={'uint8'}  byteAlign=1  blockPlatform=arduinoert
      settings: LibrarySourceBlock=mcblib/Signal Management/Byte Pack
  Constant : Constant  Value=uint8(0)
  Constant1 : Constant  Value=uint8(0)
  Constant2 : Constant  Value=hex2dec('13')  OutDataTypeStr=uint8
  Constant3 : Constant  Value=hex2dec('44')  OutDataTypeStr=uint8
  Constant4 : Constant  Value=hex2dec('13')  OutDataTypeStr=uint8
  Constant5 : Constant  Value=hex2dec('45')  OutDataTypeStr=uint8
  Constant6 : Constant  Value=8192
  Data Type Conversion : DataTypeConversion  OutDataTypeStr=double  SaturateOnIntegerOverflow=off  RndMeth=Floor
  I2C Controller Read : stm32blockslib/I2C Controller Read  I2CModule=I2C1  Mode=Controller  AddressingMode=7-bits  PeripheralByteOrder=LittleEndian  OwnPeripheralAddress=uint8(170)  PeripheralAddressVia=Inport  PeripheralAddress=0x19  RegisterAddressMode=on  RegisterAddressVia=Inport  RegisterAddress=0x02  RepeatedStart=off  NoAck=off  OutputStatus=off  BlockMode=Receive  DataType=uint8  DataLength=1  Timeout=0.001  SampleTime=-1
      settings: LibrarySourceBlock=stm32f4xxblockslib/I2C Controller Read
  I2C Controller Read4 : stm32blockslib/I2C Controller Read  I2CModule=I2C1  Mode=Controller  AddressingMode=7-bits  PeripheralByteOrder=LittleEndian  OwnPeripheralAddress=uint8(170)  PeripheralAddressVia=Inport  PeripheralAddress=0x19  RegisterAddressMode=on  RegisterAddressVia=Inport  RegisterAddress=0x02  RepeatedStart=off  NoAck=off  OutputStatus=off  BlockMode=Receive  DataType=uint8  DataLength=1  Timeout=0.001  SampleTime=-1
      settings: LibrarySourceBlock=stm32f4xxblockslib/I2C Controller Read
  Shift Arithmetic : ArithShift  BitShiftNumber=3  BitShiftDirection=Right
  Shift Arithmetic1 : ArithShift  BitShiftNumber=5  BitShiftDirection=Left
  Switch : Switch  Criteria=u2 > Threshold  Threshold=4095  SaturateOnIntegerOverflow=off  InputSameDT=off
  Vector Concatenate1 : Concatenate
  Vector Concatenate2 : Concatenate
  Out1 : Outport
  wires:
  Add/1 -> Switch/1
  Constant4/1 -> I2C Controller Read4/1
  Switch/1 -> Data Type Conversion/1
  Bitwise OR/1 -> Switch/2, Add/2, Switch/3
  Constant6/1 -> Add/1
  Constant5/1 -> I2C Controller Read4/2
  Data Type Conversion/1 -> Out1/1
  Shift Arithmetic1/1 -> Bitwise OR/2
  Vector Concatenate1/1 -> Byte Pack2/1
  Byte Pack2/1 -> Shift Arithmetic1/1
  Byte Pack1/1 -> Shift Arithmetic/1
  Vector Concatenate2/1 -> Byte Pack1/1
  Shift Arithmetic/1 -> Bitwise OR/1
  I2C Controller Read/1 -> Vector Concatenate2/1  "LSB"
  Constant2/1 -> I2C Controller Read/1
  Constant3/1 -> I2C Controller Read/2
  Constant1/1 -> Vector Concatenate2/2
  Constant/1 -> Vector Concatenate1/2
  I2C Controller Read4/1 -> Vector Concatenate1/1  "MSB"

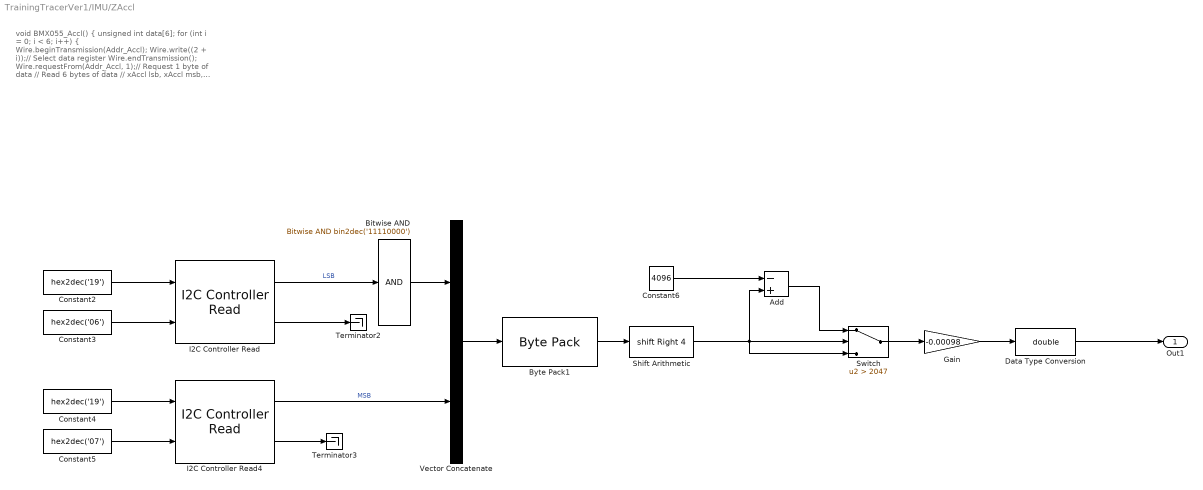
== system TrainingTracerVer1/IMU/ZAccl ==
  note: void BMX055_Accl()
      | {
      | unsigned int data[6];
      | for (int i = 0; i < 6; i++)
      | {
      | Wire.beginTransmission(Addr_Accl);
      | Wire.write((2 + i));// Select data register
      | Wire.endTransmission();
      | Wire.requestFrom(Addr_Accl, 1);// Request 1 byte of data
      | // Read 6 bytes of data
      | // xAccl lsb, xAccl msb, yAccl lsb, yAccl msb, zAccl lsb, zAccl msb
      | if (Wire.available() == 1)
      | data[i] = Wire.read();
      | }
      | // Convert the data to 12-bits
      | zAccl = ((data[5] * 256) + (data[4] & 0xF0)) / 16;
      | if (zAccl > 2047) zAccl -= 4096;
      | zAccl = zAccl * 0.00098; // range = +/-2g
      | }
  Add : Sum  Inputs=-+
  Bitwise AND : simulink/Logic and Bit Operations/Bitwise Operator  logicop=AND  UseBitMask=on  BitMask=bin2dec('11110000')  BitMaskRealWorld=Stored Integer
      settings: LibrarySourceBlock=|
      | simulink/Quick Insert/Logic and Bit
      | Operations/Bitwise AND
  Byte Pack1 : svdutilitieslib/Byte Pack  maskPackedDataType=uint16  datatypes={'uint8'}  byteAlign=1  blockPlatform=arduinoert
      settings: LibrarySourceBlock=mcblib/Signal Management/Byte Pack
  Constant2 : Constant  Value=hex2dec('19')  OutDataTypeStr=uint8
  Constant3 : Constant  Value=hex2dec('06')  OutDataTypeStr=uint8
  Constant4 : Constant  Value=hex2dec('19')  OutDataTypeStr=uint8
  Constant5 : Constant  Value=hex2dec('07')  OutDataTypeStr=uint8
  Constant6 : Constant  Value=4096
  Data Type Conversion : DataTypeConversion  OutDataTypeStr=double  SaturateOnIntegerOverflow=off  RndMeth=Floor
  Gain : Gain  Gain=-0.00098
  I2C Controller Read : stm32blockslib/I2C Controller Read  I2CModule=I2C1  Mode=Controller  AddressingMode=7-bits  PeripheralByteOrder=LittleEndian  OwnPeripheralAddress=uint8(170)  PeripheralAddressVia=Inport  PeripheralAddress=0x19  RegisterAddressMode=on  RegisterAddressVia=Inport  RegisterAddress=0x02  RepeatedStart=off  NoAck=off  OutputStatus=on  BlockMode=Receive  DataType=uint8  DataLength=1  Timeout=0.1  SampleTime=-1
      settings: LibrarySourceBlock=stm32f4xxblockslib/I2C Controller Read
  I2C Controller Read4 : stm32blockslib/I2C Controller Read  I2CModule=I2C1  Mode=Controller  AddressingMode=7-bits  PeripheralByteOrder=LittleEndian  OwnPeripheralAddress=uint8(170)  PeripheralAddressVia=Inport  PeripheralAddress=0x19  RegisterAddressMode=on  RegisterAddressVia=Inport  RegisterAddress=0x02  RepeatedStart=off  NoAck=off  OutputStatus=on  BlockMode=Receive  DataType=uint8  DataLength=1  Timeout=0.1  SampleTime=-1
      settings: LibrarySourceBlock=stm32f4xxblockslib/I2C Controller Read
  Shift Arithmetic : ArithShift  BitShiftNumber=4  BitShiftDirection=Right
  Switch : Switch  Criteria=u2 > Threshold  Threshold=2047  SaturateOnIntegerOverflow=off  InputSameDT=off
  Terminator2 : Terminator
  Terminator3 : Terminator
  Vector Concatenate : Concatenate
  Out1 : Outport
  wires:
  Constant3/1 -> I2C Controller Read/2
  Add/1 -> Switch/1
  Constant4/1 -> I2C Controller Read4/1
  Byte Pack1/1 -> Shift Arithmetic/1
  Gain/1 -> Data Type Conversion/1
  I2C Controller Read/2 -> Terminator2/1
  Constant2/1 -> I2C Controller Read/1
  Shift Arithmetic/1 -> Switch/2, Switch/3, Add/2
  Bitwise AND/1 -> Vector Concatenate/1
  Constant6/1 -> Add/1
  I2C Controller Read4/2 -> Terminator3/1
  I2C Controller Read4/1 -> Vector Concatenate/2  "MSB"
  Constant5/1 -> I2C Controller Read4/2
  Switch/1 -> Gain/1
  I2C Controller Read/1 -> Bitwise AND/1  "LSB"
  Vector Concatenate/1 -> Byte Pack1/1
  Data Type Conversion/1 -> Out1/1

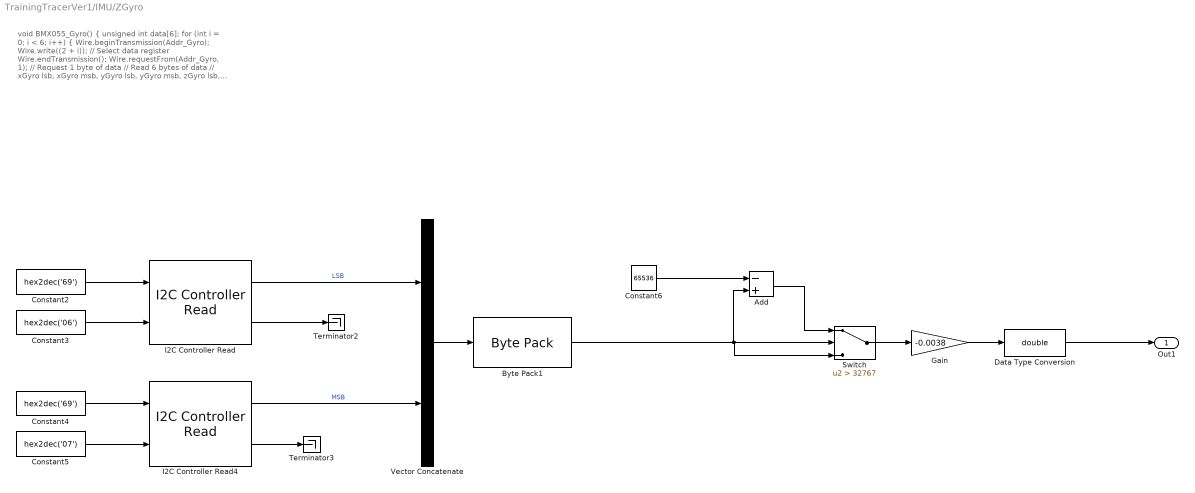
== system TrainingTracerVer1/IMU/ZGyro ==
  note: void BMX055_Gyro()
      | {
      | unsigned int data[6];
      | for (int i = 0; i < 6; i++)
      | {
      | Wire.beginTransmission(Addr_Gyro);
      | Wire.write((2 + i)); // Select data register
      | Wire.endTransmission();
      | Wire.requestFrom(Addr_Gyro, 1); // Request 1 byte of data
      | // Read 6 bytes of data
      | // xGyro lsb, xGyro msb, yGyro lsb, yGyro msb, zGyro lsb, zGyro msb
      | if (Wire.available() == 1)
      | data[i] = Wire.read();
      | }
      | // Convert the data
      | zGyro = (data[5] * 256) + data[4];
      | if (zGyro > 32767) zGyro -= 65536;
      | zGyro = zGyro * 0.0038; // Full scale = +/- 125 degree/s
      | }
  Add : Sum  Inputs=-+
  Byte Pack1 : svdutilitieslib/Byte Pack  maskPackedDataType=uint16  datatypes={'uint8'}  byteAlign=1  blockPlatform=arduinoert
      settings: LibrarySourceBlock=mcblib/Signal Management/Byte Pack
  Constant2 : Constant  Value=hex2dec('69')  OutDataTypeStr=uint8
  Constant3 : Constant  Value=hex2dec('06')  OutDataTypeStr=uint8
  Constant4 : Constant  Value=hex2dec('69')  OutDataTypeStr=uint8
  Constant5 : Constant  Value=hex2dec('07')  OutDataTypeStr=uint8
  Constant6 : Constant  Value=65536
  Data Type Conversion : DataTypeConversion  OutDataTypeStr=double  SaturateOnIntegerOverflow=off  RndMeth=Floor
  Gain : Gain  Gain=-0.0038
  I2C Controller Read : stm32blockslib/I2C Controller Read  I2CModule=I2C1  Mode=Controller  AddressingMode=7-bits  PeripheralByteOrder=LittleEndian  OwnPeripheralAddress=uint8(170)  PeripheralAddressVia=Inport  PeripheralAddress=0x19  RegisterAddressMode=on  RegisterAddressVia=Inport  RegisterAddress=0x02  RepeatedStart=off  NoAck=off  OutputStatus=on  BlockMode=Receive  DataType=uint8  DataLength=1  Timeout=0.001  SampleTime=-1
      settings: LibrarySourceBlock=stm32f4xxblockslib/I2C Controller Read
  I2C Controller Read4 : stm32blockslib/I2C Controller Read  I2CModule=I2C1  Mode=Controller  AddressingMode=7-bits  PeripheralByteOrder=LittleEndian  OwnPeripheralAddress=uint8(170)  PeripheralAddressVia=Inport  PeripheralAddress=0x19  RegisterAddressMode=on  RegisterAddressVia=Inport  RegisterAddress=0x02  RepeatedStart=off  NoAck=off  OutputStatus=on  BlockMode=Receive  DataType=uint8  DataLength=1  Timeout=0.001  SampleTime=-1
      settings: LibrarySourceBlock=stm32f4xxblockslib/I2C Controller Read
  Switch : Switch  Criteria=u2 > Threshold  Threshold=32767  SaturateOnIntegerOverflow=off  InputSameDT=off
  Terminator2 : Terminator
  Terminator3 : Terminator
  Vector Concatenate : Concatenate
  Out1 : Outport
  wires:
  Constant3/1 -> I2C Controller Read/2
  Add/1 -> Switch/1
  Constant4/1 -> I2C Controller Read4/1
  Gain/1 -> Data Type Conversion/1
  I2C Controller Read/2 -> Terminator2/1
  Constant2/1 -> I2C Controller Read/1
  Byte Pack1/1 -> Switch/2, Switch/3, Add/2
  Constant6/1 -> Add/1
  I2C Controller Read4/2 -> Terminator3/1
  I2C Controller Read4/1 -> Vector Concatenate/2  "MSB"
  Constant5/1 -> I2C Controller Read4/2
  Switch/1 -> Gain/1
  I2C Controller Read/1 -> Vector Concatenate/1  "LSB"
  Vector Concatenate/1 -> Byte Pack1/1
  Data Type Conversion/1 -> Out1/1
